simulink model "speed_verification_system"  (R2024a)
settings: Solver=VariableStepAuto  StartTime=0.0  StopTime=inf  RelTol=1e-3
libraries: simulink x4
settings Model: Creator=admin  LastModifiedBy=admin

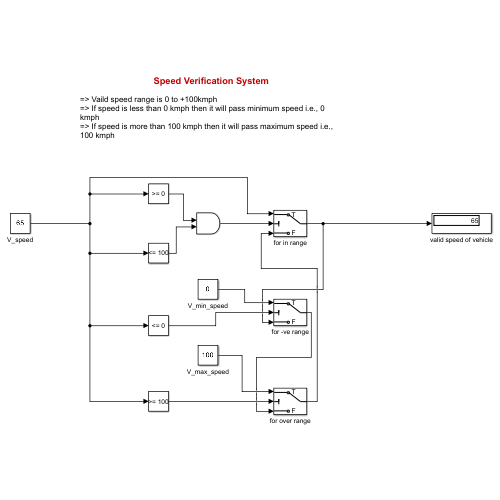
[thumbnail: Simulink's stored preview of the top-level diagram]
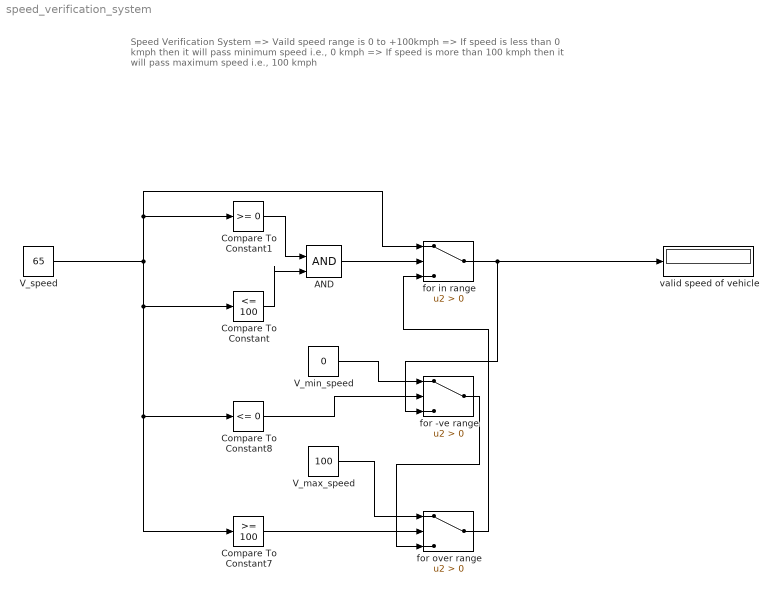
== system speed_verification_system ==
  note: Speed Verification System
      |
      | => Vaild speed range is 0 to +100kmph
      | => If speed is less than 0 kmph then it will pass minimum speed i.e., 0 kmph
      | => If speed is more than 100 kmph then it will pass maximum speed i.e., 100 kmph
  AND : Logic  IconShape=distinctive  AllPortsSameDT=off  OutDataTypeStr=boolean
  Compare To Constant : simulink/Logic and Bit Operations/Compare To Constant  relop=<=  const=100  OutDataTypeStr=boolean
  Compare To Constant1 : simulink/Logic and Bit Operations/Compare To Constant  relop=>=  const=0  OutDataTypeStr=boolean
  Compare To Constant7 : simulink/Logic and Bit Operations/Compare To Constant  relop=>=  const=100  OutDataTypeStr=boolean
  Compare To Constant8 : simulink/Logic and Bit Operations/Compare To Constant  relop=<=  const=0  OutDataTypeStr=boolean
  V_max_speed : Constant  Value=100
  V_min_speed : Constant  Value=0
  V_speed : Constant  Value=65
  for -ve range : Switch  Criteria=u2 > Threshold  SaturateOnIntegerOverflow=off  InputSameDT=off
  for in range : Switch  Criteria=u2 > Threshold  SaturateOnIntegerOverflow=off  InputSameDT=off
  for over range : Switch  Criteria=u2 > Threshold  SaturateOnIntegerOverflow=off  InputSameDT=off
  valid speed of vehicle : Display
  wires:
  Compare To Constant1/1 -> AND/1
  Compare To Constant/1 -> AND/2
  V_speed/1 -> Compare To Constant1/1, for in range/1, Compare To Constant7/1, Compare To Constant8/1, Compare To Constant/1
  Compare To Constant8/1 -> for -ve range/2
  V_min_speed/1 -> for -ve range/1
  AND/1 -> for in range/2
  for in range/1 -> for -ve range/3, valid speed of vehicle/1
  Compare To Constant7/1 -> for over range/2
  V_max_speed/1 -> for over range/1
  for -ve range/1 -> for over range/3
  for over range/1 -> for in range/3
